simulink model "control_demo"  (R2022a)
settings: Solver=FixedStepAuto  StartTime=0.0  StopTime=10  FixedStep=Ts  RelTol=1e-3
values from neighbouring files (symbols this model uses):
  fil = 0.1    [Decen_control_prepare.m]    (also in control_demo_prepare.m = 0.0001; simulation_CPG.m = 0.0001)
  K_a = diag([0.001,0.001])    [control_demo_prepare.m]
  K_d = diag([5,5])    [control_demo_prepare.m]    (also in simulation_CPG.m)
  K_p = diag([1000,1000])    [control_demo_prepare.m]    (also in simulation_CPG.m)
  Tc = 0.001    [Decen_control_prepare.m]    (also in control_demo_prepare.m; simulation_CPG.m)
undefined symbols (not defined in the file or in its folder): duration, effort, IFV, index, iner, joint_name, LF_body2thigh, LF_thigh2calf, LH_body2thigh, LH_thigh2calf, model_name, RF_body2thigh, RF_thigh2calf, RH_body2thigh, RH_thigh2calf
libraries: robotgazebolib x27
settings Model: PauseTimes=2  Creator=liltrump  LastModifiedBy=liltrump

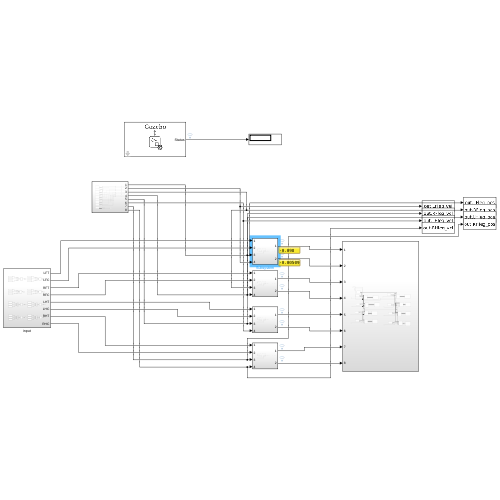
[thumbnail: Simulink's stored preview of the top-level diagram]
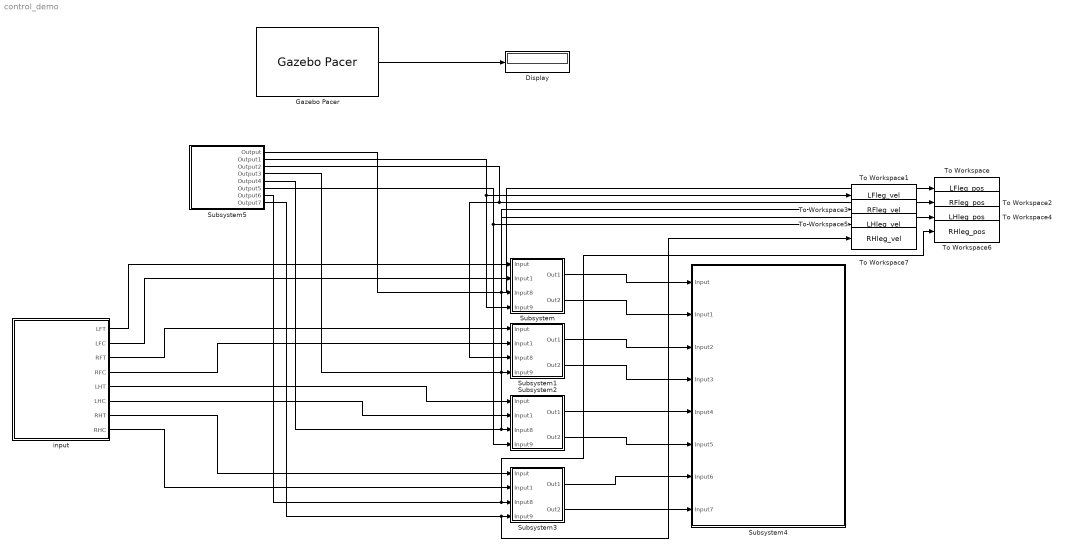
== system control_demo ==
  Display : Display
  Gazebo Pacer : robotgazebolib/Gazebo Pacer  ResetBehavior=Reset Gazebo simulation time and scene  SampleTime=0.001
      settings: SourceProductBaseCode=RO
  Subsystem : Subsystem
  Subsystem1 : Subsystem
  Subsystem2 : Subsystem
  Subsystem3 : Subsystem
  Subsystem4 : Subsystem
  Subsystem5 : Subsystem
  To Workspace : ToWorkspace  VariableName=LFleg_pos  SaveFormat=Timeseries  SampleTime=-1
  To Workspace1 : ToWorkspace  VariableName=LFleg_vel  SaveFormat=Timeseries  SampleTime=-1
  To Workspace2 : ToWorkspace  VariableName=RFleg_pos  SaveFormat=Timeseries  SampleTime=-1
  To Workspace3 : ToWorkspace  VariableName=RFleg_vel  SaveFormat=Timeseries  SampleTime=-1
  To Workspace4 : ToWorkspace  VariableName=LHleg_pos  SaveFormat=Timeseries  SampleTime=-1
  To Workspace5 : ToWorkspace  VariableName=LHleg_vel  SaveFormat=Timeseries  SampleTime=-1
  To Workspace6 : ToWorkspace  VariableName=RHleg_pos  SaveFormat=Timeseries  SampleTime=-1
  To Workspace7 : ToWorkspace  VariableName=RHleg_vel  SaveFormat=Timeseries  SampleTime=-1
  input : Subsystem
  wires:
  Gazebo Pacer/1 -> Display/1
  Subsystem5/1(Output) -> To Workspace/1, Subsystem/3(Input8)
  Subsystem5/2(Output1) -> To Workspace1/1, Subsystem/4(Input9)
  Subsystem5/3(Output2) -> Subsystem1/3(Input8), To Workspace2/1
  Subsystem5/4(Output3) -> Subsystem1/4(Input9), To Workspace3/1
  Subsystem5/5(Output4) -> Subsystem2/3(Input8), To Workspace4/1
  Subsystem5/6(Output5) -> Subsystem2/4(Input9), To Workspace5/1
  Subsystem5/7(Output6) -> Subsystem3/3(Input8), To Workspace6/1
  Subsystem5/8(Output7) -> Subsystem3/4(Input9), To Workspace7/1
  Subsystem/1(Out1) -> Subsystem4/1(Input)
  Subsystem/2(Out2) -> Subsystem4/2(Input1)
  Subsystem1/1(Out1) -> Subsystem4/3(Input2)
  Subsystem1/2(Out2) -> Subsystem4/4(Input3)
  Subsystem2/1(Out1) -> Subsystem4/5(Input4)
  Subsystem2/2(Out2) -> Subsystem4/6(Input5)
  Subsystem3/1(Out1) -> Subsystem4/7(Input6)
  Subsystem3/2(Out2) -> Subsystem4/8(Input7)
  input/1(LFT) -> Subsystem/1(Input)
  input/2(LFC) -> Subsystem/2(Input1)
  input/3(RFT) -> Subsystem1/1(Input)
  input/4(RFC) -> Subsystem1/2(Input1)
  input/5(LHT) -> Subsystem2/1(Input)
  input/6(LHC) -> Subsystem2/2(Input1)
  input/7(RHT) -> Subsystem3/1(Input)
  input/8(RHC) -> Subsystem3/2(Input1)

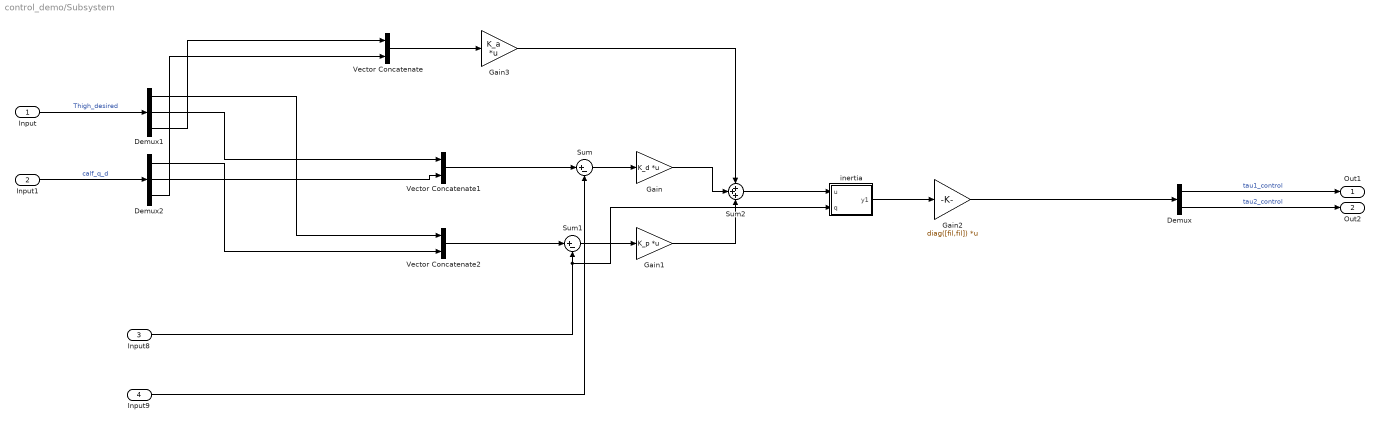
== system control_demo/Subsystem ==
  Input : Inport
  Input1 : Inport  Port=2
  Input8 : Inport  Port=3
  Input9 : Inport  Port=4
  Demux : Demux  Outputs=2
  Demux1 : Demux  Outputs=3
  Demux2 : Demux  Outputs=3
  Gain : Gain  Gain=K_d  Multiplication=Matrix(K*u)
  Gain1 : Gain  Gain=K_p  Multiplication=Matrix(K*u)
  Gain2 : Gain  Gain=diag([fil,fil])  Multiplication=Matrix(K*u)
  Gain3 : Gain  Gain=K_a  Multiplication=Matrix(K*u)
  Sum : Sum  Inputs=|+-
  Sum1 : Sum  Inputs=|+-
  Sum2 : Sum  Inputs=+++
  Vector Concatenate : Concatenate
  Vector Concatenate1 : Concatenate
  Vector Concatenate2 : Concatenate
  inertia : Subsystem
      mask Display: disp('B(q)u')
  Out1 : Outport
  Out2 : Outport  Port=2
  wires:
  Gain1/1 -> Sum2/3
  Vector Concatenate1/1 -> Sum/1
  Sum/1 -> Gain/1
  Sum2/1 -> inertia/1(u)
  Sum1/1 -> Gain1/1
  Gain/1 -> Sum2/2
  Vector Concatenate2/1 -> Sum1/1
  Input8/1 -> inertia/2(q), Sum1/2
  Input9/1 -> Sum/2
  Demux/2 -> Out2/1  "tau2_control"
  Demux/1 -> Out1/1  "tau1_control"
  inertia/1(y1) -> Gain2/1
  Gain2/1 -> Demux/1
  Input/1 -> Demux1/1  "Thigh_desired"
  Input1/1 -> Demux2/1  "calf_q_d"
  Demux1/1 -> Vector Concatenate2/1
  Demux2/1 -> Vector Concatenate2/2
  Demux1/2 -> Vector Concatenate1/1
  Demux2/2 -> Vector Concatenate1/2
  Demux1/3 -> Vector Concatenate/1
  Demux2/3 -> Vector Concatenate/2
  Vector Concatenate/1 -> Gain3/1
  Gain3/1 -> Sum2/1

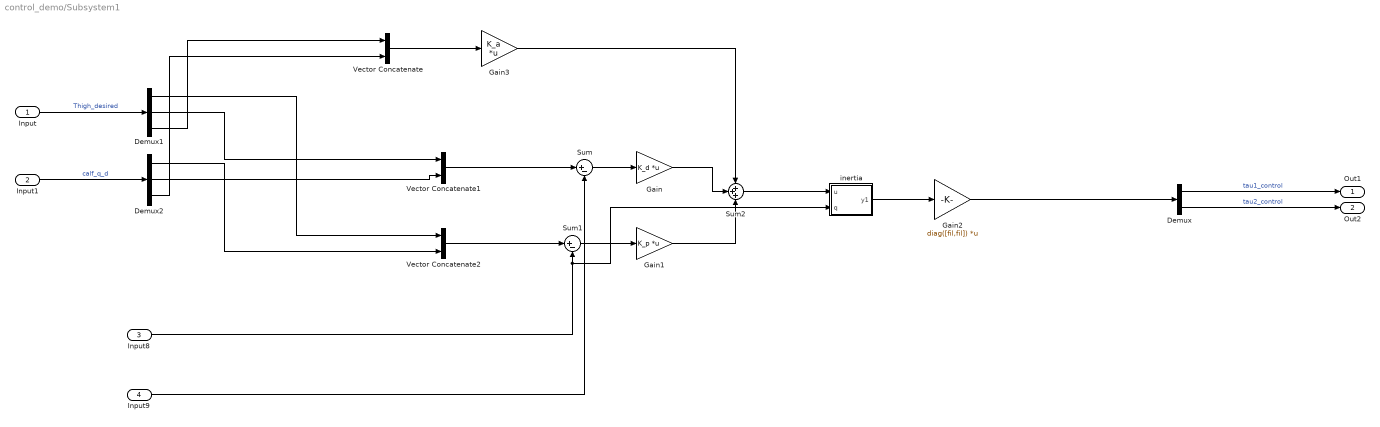
== system control_demo/Subsystem1 ==
  Input : Inport
  Input1 : Inport  Port=2
  Input8 : Inport  Port=3
  Input9 : Inport  Port=4
  Demux : Demux  Outputs=2
  Demux1 : Demux  Outputs=3
  Demux2 : Demux  Outputs=3
  Gain : Gain  Gain=K_d  Multiplication=Matrix(K*u)
  Gain1 : Gain  Gain=K_p  Multiplication=Matrix(K*u)
  Gain2 : Gain  Gain=diag([fil,fil])  Multiplication=Matrix(K*u)
  Gain3 : Gain  Gain=K_a  Multiplication=Matrix(K*u)
  Sum : Sum  Inputs=|+-
  Sum1 : Sum  Inputs=|+-
  Sum2 : Sum  Inputs=+++
  Vector Concatenate : Concatenate
  Vector Concatenate1 : Concatenate
  Vector Concatenate2 : Concatenate
  inertia : Subsystem
      mask Display: disp('B(q)u')
  Out1 : Outport
  Out2 : Outport  Port=2
  wires:
  Gain1/1 -> Sum2/3
  Vector Concatenate1/1 -> Sum/1
  Sum/1 -> Gain/1
  Sum2/1 -> inertia/1(u)
  Sum1/1 -> Gain1/1
  Gain/1 -> Sum2/2
  Vector Concatenate2/1 -> Sum1/1
  Input8/1 -> inertia/2(q), Sum1/2
  Input9/1 -> Sum/2
  Demux/2 -> Out2/1  "tau2_control"
  Demux/1 -> Out1/1  "tau1_control"
  inertia/1(y1) -> Gain2/1
  Gain2/1 -> Demux/1
  Input/1 -> Demux1/1  "Thigh_desired"
  Input1/1 -> Demux2/1  "calf_q_d"
  Demux1/1 -> Vector Concatenate2/1
  Demux2/1 -> Vector Concatenate2/2
  Demux1/2 -> Vector Concatenate1/1
  Demux2/2 -> Vector Concatenate1/2
  Demux1/3 -> Vector Concatenate/1
  Demux2/3 -> Vector Concatenate/2
  Vector Concatenate/1 -> Gain3/1
  Gain3/1 -> Sum2/1

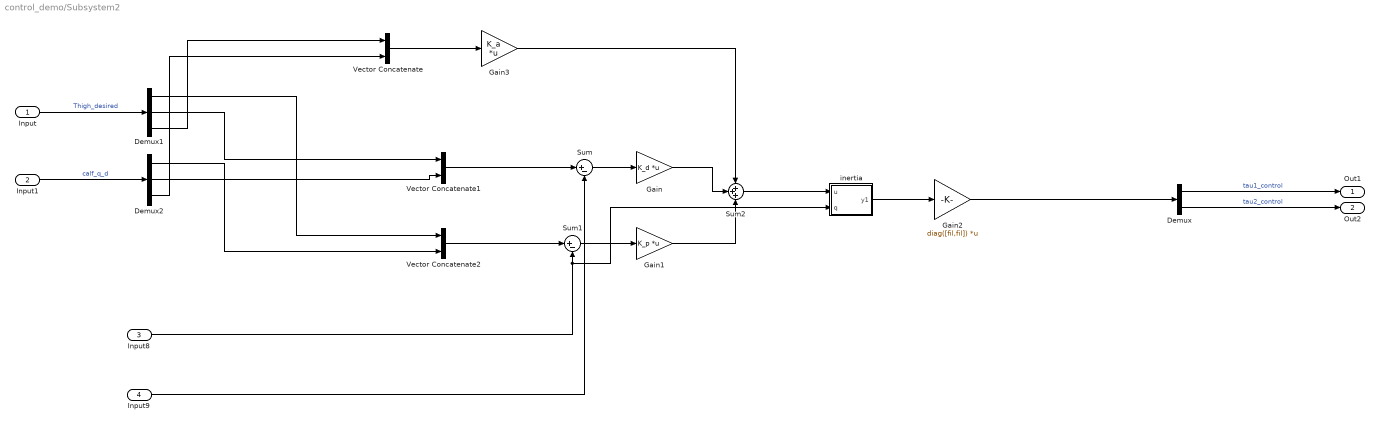
== system control_demo/Subsystem2 ==
  Input : Inport
  Input1 : Inport  Port=2
  Input8 : Inport  Port=3
  Input9 : Inport  Port=4
  Demux : Demux  Outputs=2
  Demux1 : Demux  Outputs=3
  Demux2 : Demux  Outputs=3
  Gain : Gain  Gain=K_d  Multiplication=Matrix(K*u)
  Gain1 : Gain  Gain=K_p  Multiplication=Matrix(K*u)
  Gain2 : Gain  Gain=diag([fil,fil])  Multiplication=Matrix(K*u)
  Gain3 : Gain  Gain=K_a  Multiplication=Matrix(K*u)
  Sum : Sum  Inputs=|+-
  Sum1 : Sum  Inputs=|+-
  Sum2 : Sum  Inputs=+++
  Vector Concatenate : Concatenate
  Vector Concatenate1 : Concatenate
  Vector Concatenate2 : Concatenate
  inertia : Subsystem
      mask Display: disp('B(q)u')
  Out1 : Outport
  Out2 : Outport  Port=2
  wires:
  Gain1/1 -> Sum2/3
  Vector Concatenate1/1 -> Sum/1
  Sum/1 -> Gain/1
  Sum2/1 -> inertia/1(u)
  Sum1/1 -> Gain1/1
  Gain/1 -> Sum2/2
  Vector Concatenate2/1 -> Sum1/1
  Input8/1 -> inertia/2(q), Sum1/2
  Input9/1 -> Sum/2
  Demux/2 -> Out2/1  "tau2_control"
  Demux/1 -> Out1/1  "tau1_control"
  inertia/1(y1) -> Gain2/1
  Gain2/1 -> Demux/1
  Input/1 -> Demux1/1  "Thigh_desired"
  Input1/1 -> Demux2/1  "calf_q_d"
  Demux1/1 -> Vector Concatenate2/1
  Demux2/1 -> Vector Concatenate2/2
  Demux1/2 -> Vector Concatenate1/1
  Demux2/2 -> Vector Concatenate1/2
  Demux1/3 -> Vector Concatenate/1
  Demux2/3 -> Vector Concatenate/2
  Vector Concatenate/1 -> Gain3/1
  Gain3/1 -> Sum2/1

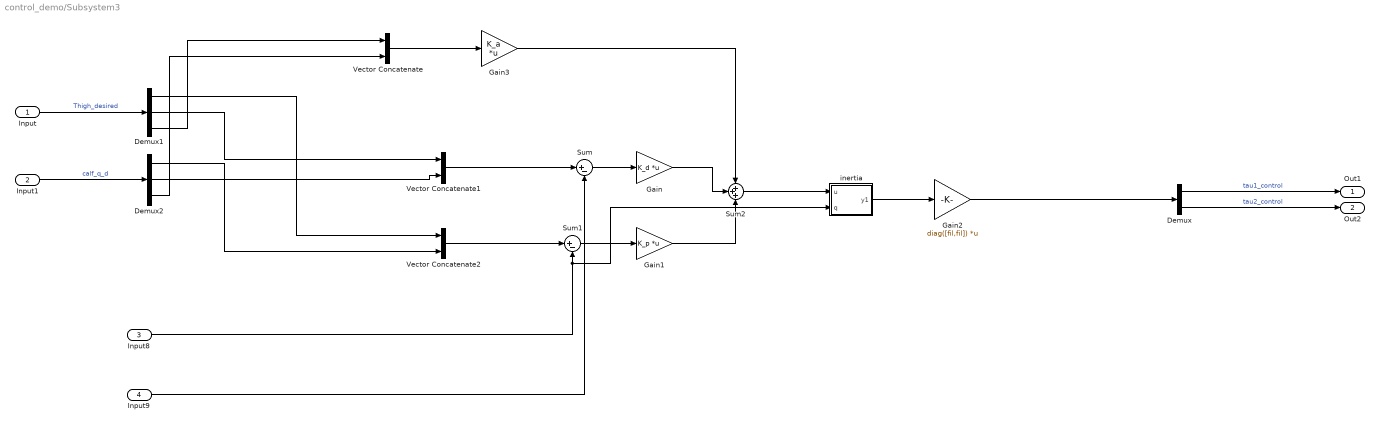
== system control_demo/Subsystem3 ==
  Input : Inport
  Input1 : Inport  Port=2
  Input8 : Inport  Port=3
  Input9 : Inport  Port=4
  Demux : Demux  Outputs=2
  Demux1 : Demux  Outputs=3
  Demux2 : Demux  Outputs=3
  Gain : Gain  Gain=K_d  Multiplication=Matrix(K*u)
  Gain1 : Gain  Gain=K_p  Multiplication=Matrix(K*u)
  Gain2 : Gain  Gain=diag([fil,fil])  Multiplication=Matrix(K*u)
  Gain3 : Gain  Gain=K_a  Multiplication=Matrix(K*u)
  Sum : Sum  Inputs=|+-
  Sum1 : Sum  Inputs=|+-
  Sum2 : Sum  Inputs=+++
  Vector Concatenate : Concatenate
  Vector Concatenate1 : Concatenate
  Vector Concatenate2 : Concatenate
  inertia : Subsystem
      mask Display: disp('B(q)u')
  Out1 : Outport
  Out2 : Outport  Port=2
  wires:
  Gain1/1 -> Sum2/3
  Vector Concatenate1/1 -> Sum/1
  Sum/1 -> Gain/1
  Sum2/1 -> inertia/1(u)
  Sum1/1 -> Gain1/1
  Gain/1 -> Sum2/2
  Vector Concatenate2/1 -> Sum1/1
  Input8/1 -> inertia/2(q), Sum1/2
  Input9/1 -> Sum/2
  Demux/2 -> Out2/1  "tau2_control"
  Demux/1 -> Out1/1  "tau1_control"
  inertia/1(y1) -> Gain2/1
  Gain2/1 -> Demux/1
  Input/1 -> Demux1/1  "Thigh_desired"
  Input1/1 -> Demux2/1  "calf_q_d"
  Demux1/1 -> Vector Concatenate2/1
  Demux2/1 -> Vector Concatenate2/2
  Demux1/2 -> Vector Concatenate1/1
  Demux2/2 -> Vector Concatenate1/2
  Demux1/3 -> Vector Concatenate/1
  Demux2/3 -> Vector Concatenate/2
  Vector Concatenate/1 -> Gain3/1
  Gain3/1 -> Sum2/1

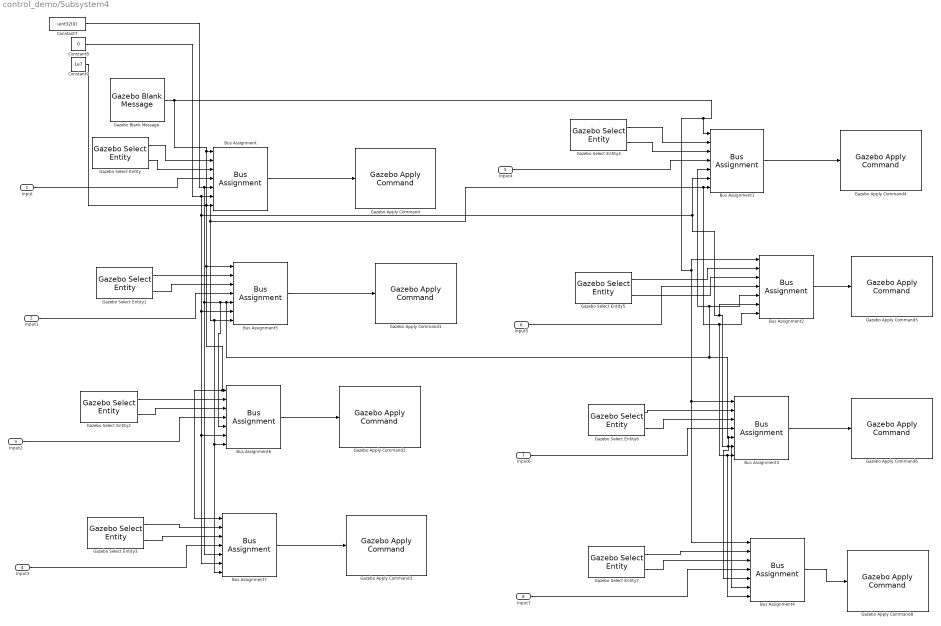
== system control_demo/Subsystem4 ==
  Input : Inport
  Input1 : Inport  Port=2
  Input2 : Inport  Port=3
  Input3 : Inport  Port=4
  Input4 : Inport  Port=5
  Input5 : Inport  Port=6
  Input6 : Inport  Port=7
  Input7 : Inport  Port=8
  Bus Assignment{,1..7} (8 alike) : BusAssignment  AssignedSignals=model_name,joint_name,effort,index,duration.seconds,duration.nano_seconds
  Constant7 : Constant  Value=uint32(0)
  Constant8 : Constant  Value=0
  Constant9 : Constant  Value=1e7
  Gazebo Apply Command{,1..6,8} (8 alike) : robotgazebolib/Gazebo Apply Command  cmdType=ApplyJointTorque  sampleTime=0.001
      settings: SourceProductBaseCode=RO
  Gazebo Blank Message : robotgazebolib/Gazebo Blank Message  msgType=ApplyJointTorque  sampleTime=0.001  busName='Gazebo_SL_Bus_gazebo_msgs_ApplyJointTorque'
      settings: SourceProductBaseCode=RO
  Gazebo Select Entity : robotgazebolib/Gazebo Select Entity  modelElemName=IFV/LF_body2thigh  outputArraySize=128  OutputLabel=Joint  SelectType=Joint
      settings: SourceProductBaseCode=RO
  Gazebo Select Entity1 : robotgazebolib/Gazebo Select Entity  modelElemName=IFV/LF_thigh2calf  outputArraySize=128  OutputLabel=Joint  SelectType=Joint
      settings: SourceProductBaseCode=RO
  Gazebo Select Entity2 : robotgazebolib/Gazebo Select Entity  modelElemName=IFV/RF_body2thigh  outputArraySize=128  OutputLabel=Joint  SelectType=Joint
      settings: SourceProductBaseCode=RO
  Gazebo Select Entity3 : robotgazebolib/Gazebo Select Entity  modelElemName=IFV/RF_thigh2calf  outputArraySize=128  OutputLabel=Joint  SelectType=Joint
      settings: SourceProductBaseCode=RO
  Gazebo Select Entity4 : robotgazebolib/Gazebo Select Entity  modelElemName=IFV/LH_body2thigh  outputArraySize=128  OutputLabel=Joint  SelectType=Joint
      settings: SourceProductBaseCode=RO
  Gazebo Select Entity5 : robotgazebolib/Gazebo Select Entity  modelElemName=IFV/LH_thigh2calf  outputArraySize=128  OutputLabel=Joint  SelectType=Joint
      settings: SourceProductBaseCode=RO
  Gazebo Select Entity6 : robotgazebolib/Gazebo Select Entity  modelElemName=IFV/RH_body2thigh  outputArraySize=128  OutputLabel=Joint  SelectType=Joint
      settings: SourceProductBaseCode=RO
  Gazebo Select Entity7 : robotgazebolib/Gazebo Select Entity  modelElemName=IFV/RH_thigh2calf  outputArraySize=128  OutputLabel=Joint  SelectType=Joint
      settings: SourceProductBaseCode=RO
  wires:
  Gazebo Select Entity/1 -> Bus Assignment/2
  Gazebo Select Entity/2 -> Bus Assignment/3
  Bus Assignment/1 -> Gazebo Apply Command/1
  Input/1 -> Bus Assignment/4
  Bus Assignment5/1 -> Gazebo Apply Command1/1
  Input1/1 -> Bus Assignment5/4
  Gazebo Select Entity1/1 -> Bus Assignment5/2
  Gazebo Select Entity1/2 -> Bus Assignment5/3
  Bus Assignment6/1 -> Gazebo Apply Command2/1
  Input2/1 -> Bus Assignment6/4
  Gazebo Select Entity2/1 -> Bus Assignment6/2
  Gazebo Select Entity2/2 -> Bus Assignment6/3
  Bus Assignment7/1 -> Gazebo Apply Command3/1
  Input3/1 -> Bus Assignment7/4
  Gazebo Select Entity3/1 -> Bus Assignment7/2
  Gazebo Select Entity3/2 -> Bus Assignment7/3
  Bus Assignment1/1 -> Gazebo Apply Command4/1
  Gazebo Select Entity4/1 -> Bus Assignment1/2
  Gazebo Select Entity4/2 -> Bus Assignment1/3
  Bus Assignment2/1 -> Gazebo Apply Command5/1
  Gazebo Select Entity5/1 -> Bus Assignment2/2
  Gazebo Select Entity5/2 -> Bus Assignment2/3
  Bus Assignment3/1 -> Gazebo Apply Command6/1
  Input6/1 -> Bus Assignment3/4
  Gazebo Select Entity6/1 -> Bus Assignment3/2
  Gazebo Select Entity6/2 -> Bus Assignment3/3
  Bus Assignment4/1 -> Gazebo Apply Command8/1
  Input7/1 -> Bus Assignment4/4
  Gazebo Select Entity7/1 -> Bus Assignment4/2
  Gazebo Blank Message/1 -> Bus Assignment1/1, Bus Assignment2/1, Bus Assignment4/1, Bus Assignment3/1, Bus Assignment5/1, Bus Assignment7/1, Bus Assignment6/1, Bus Assignment/1
  Gazebo Select Entity7/2 -> Bus Assignment4/3
  Constant7/1 -> Bus Assignment/5, Bus Assignment6/5, Bus Assignment4/5, Bus Assignment3/5, Bus Assignment1/5, Bus Assignment2/5, Bus Assignment5/5, Bus Assignment7/5
  Constant8/1 -> Bus Assignment7/6, Bus Assignment6/6, Bus Assignment5/6, Bus Assignment4/6, Bus Assignment3/6, Bus Assignment2/6, Bus Assignment1/6, Bus Assignment/6
  Constant9/1 -> Bus Assignment5/7, Bus Assignment7/7, Bus Assignment6/7, Bus Assignment4/7, Bus Assignment3/7, Bus Assignment2/7, Bus Assignment1/7, Bus Assignment/7
  Input4/1 -> Bus Assignment1/4
  Input5/1 -> Bus Assignment2/4

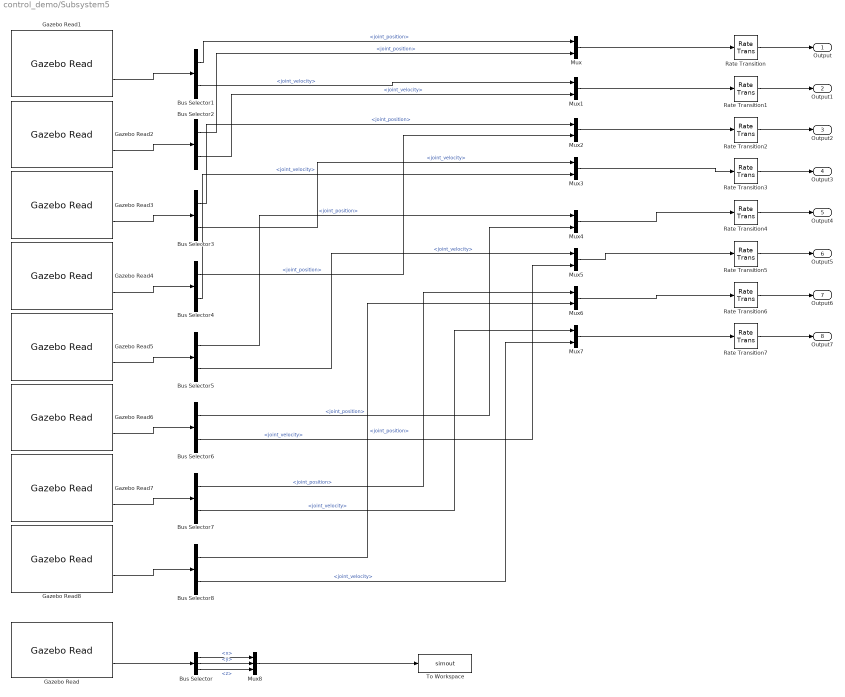
== system control_demo/Subsystem5 ==
  Bus Selector : BusSelector  OutputSignals=world_linear_velocity.x,world_linear_velocity.y,world_linear_velocity.z
  Bus Selector{1..8} (8 alike) : BusSelector  OutputSignals=joint_position,joint_velocity
  Gazebo Read : robotgazebolib/Gazebo Read  topicSource=From Gazebo  topic=/gazebo/ground_truth/link_state/IFV/chassis  messageType=gazebo_msgs/LinkState  sampleTime=0.001
      settings: SourceProductBaseCode=RO
  Gazebo Read1 : robotgazebolib/Gazebo Read  topicSource=From Gazebo  topic=/gazebo/ground_truth/joint_state/IFV/LF_body2thigh  messageType=gazebo_msgs/JointState  sampleTime=0.001
      settings: SourceProductBaseCode=RO
  Gazebo Read2 : robotgazebolib/Gazebo Read  topicSource=From Gazebo  topic=/gazebo/ground_truth/joint_state/IFV/LF_thigh2calf  messageType=gazebo_msgs/JointState  sampleTime=0.001
      settings: SourceProductBaseCode=RO
  Gazebo Read3 : robotgazebolib/Gazebo Read  topicSource=From Gazebo  topic=/gazebo/ground_truth/joint_state/IFV/RF_body2thigh  messageType=gazebo_msgs/JointState  sampleTime=0.001
      settings: SourceProductBaseCode=RO
  Gazebo Read4 : robotgazebolib/Gazebo Read  topicSource=From Gazebo  topic=/gazebo/ground_truth/joint_state/IFV/RF_thigh2calf  messageType=gazebo_msgs/JointState  sampleTime=0.001
      settings: SourceProductBaseCode=RO
  Gazebo Read5 : robotgazebolib/Gazebo Read  topicSource=From Gazebo  topic=/gazebo/ground_truth/joint_state/IFV/LH_body2thigh  messageType=gazebo_msgs/JointState  sampleTime=0.001
      settings: SourceProductBaseCode=RO
  Gazebo Read6 : robotgazebolib/Gazebo Read  topicSource=From Gazebo  topic=/gazebo/ground_truth/joint_state/IFV/LH_thigh2calf  messageType=gazebo_msgs/JointState  sampleTime=0.001
      settings: SourceProductBaseCode=RO
  Gazebo Read7 : robotgazebolib/Gazebo Read  topicSource=From Gazebo  topic=/gazebo/ground_truth/joint_state/IFV/RH_body2thigh  messageType=gazebo_msgs/JointState  sampleTime=0.001
      settings: SourceProductBaseCode=RO
  Gazebo Read8 : robotgazebolib/Gazebo Read  topicSource=From Gazebo  topic=/gazebo/ground_truth/joint_state/IFV/RH_thigh2calf  messageType=gazebo_msgs/JointState  sampleTime=0.001
      settings: SourceProductBaseCode=RO
  Mux{,1..7} (8 alike) : Mux  Inputs=2
  Mux8 : Mux  Inputs=3
  Rate Transition{,1..7} (8 alike) : RateTransition
  To Workspace : ToWorkspace  VariableName=simout  SaveFormat=Timeseries  SampleTime=-1
  Output : Outport
  Output1 : Outport  Port=2
  Output2 : Outport  Port=3
  Output3 : Outport  Port=4
  Output4 : Outport  Port=5
  Output5 : Outport  Port=6
  Output6 : Outport  Port=7
  Output7 : Outport  Port=8
  wires:
  Gazebo Read1/2 -> Bus Selector1/1
  Bus Selector2/2 -> Mux1/2  "<joint_velocity>"
  Gazebo Read2/2 -> Bus Selector2/1
  Gazebo Read3/2 -> Bus Selector3/1
  Gazebo Read4/2 -> Bus Selector4/1
  Gazebo Read5/2 -> Bus Selector5/1
  Gazebo Read6/2 -> Bus Selector6/1
  Gazebo Read7/2 -> Bus Selector7/1
  Gazebo Read8/2 -> Bus Selector8/1
  Mux1/1 -> Rate Transition1/1
  Mux2/1 -> Rate Transition2/1
  Mux3/1 -> Rate Transition3/1
  Mux4/1 -> Rate Transition4/1
  Mux5/1 -> Rate Transition5/1
  Mux6/1 -> Rate Transition6/1
  Mux7/1 -> Rate Transition7/1
  Bus Selector1/2 -> Mux1/1  "<joint_velocity>"
  Bus Selector1/1 -> Mux/1  "<joint_position>"
  Bus Selector2/1 -> Mux/2  "<joint_position>"
  Mux/1 -> Rate Transition/1
  Rate Transition/1 -> Output/1
  Rate Transition1/1 -> Output1/1
  Rate Transition2/1 -> Output2/1
  Rate Transition3/1 -> Output3/1
  Rate Transition4/1 -> Output4/1
  Rate Transition5/1 -> Output5/1
  Rate Transition6/1 -> Output6/1
  Rate Transition7/1 -> Output7/1
  Bus Selector3/1 -> Mux2/1  "<joint_position>"
  Bus Selector4/1 -> Mux2/2  "<joint_position>"
  Bus Selector3/2 -> Mux3/1  "<joint_velocity>"
  Bus Selector4/2 -> Mux3/2  "<joint_velocity>"
  Bus Selector5/1 -> Mux4/1  "<joint_position>"
  Bus Selector6/1 -> Mux4/2  "<joint_position>"
  Bus Selector5/2 -> Mux5/1  "<joint_velocity>"
  Bus Selector6/2 -> Mux5/2  "<joint_velocity>"
  Bus Selector7/1 -> Mux6/1  "<joint_position>"
  Bus Selector7/2 -> Mux7/1  "<joint_velocity>"
  Bus Selector8/1 -> Mux6/2  "<joint_position>"
  Bus Selector8/2 -> Mux7/2  "<joint_velocity>"
  Gazebo Read/2 -> Bus Selector/1
  Bus Selector/1 -> Mux8/1  "<x>"
  Bus Selector/3 -> Mux8/3  "<z>"
  Mux8/1 -> To Workspace/1
  Bus Selector/2 -> Mux8/2  "<y>"

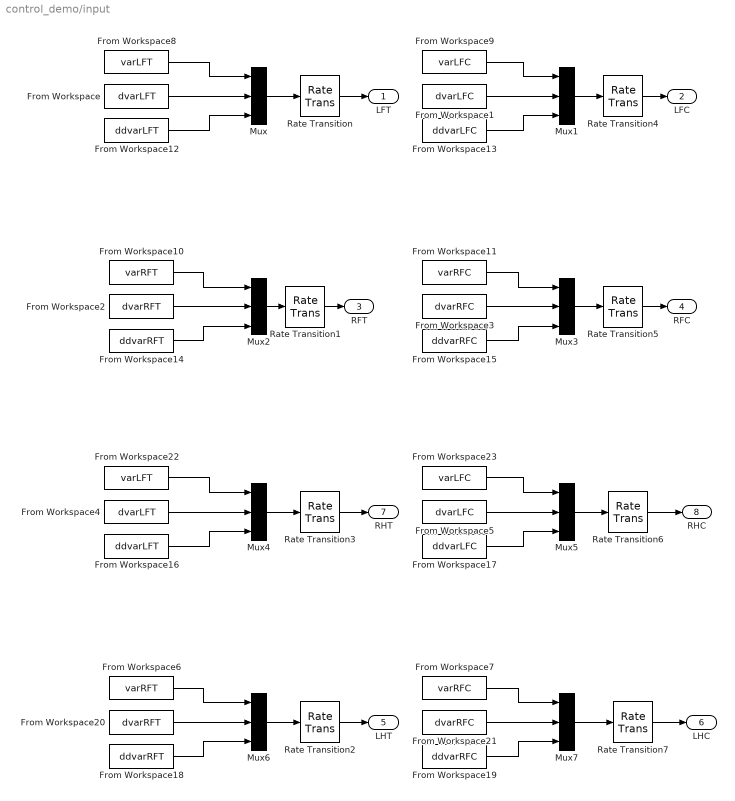
== system control_demo/input ==
  From Workspace : FromWorkspace  VariableName=dvarLFT
  From Workspace1 : FromWorkspace  VariableName=dvarLFC
  From Workspace10 : FromWorkspace  VariableName=varRFT
  From Workspace11 : FromWorkspace  VariableName=varRFC
  From Workspace12 : FromWorkspace  VariableName=ddvarLFT
  From Workspace13 : FromWorkspace  VariableName=ddvarLFC
  From Workspace14 : FromWorkspace  VariableName=ddvarRFT
  From Workspace15 : FromWorkspace  VariableName=ddvarRFC
  From Workspace16 : FromWorkspace  VariableName=ddvarLFT
  From Workspace17 : FromWorkspace  VariableName=ddvarLFC
  From Workspace18 : FromWorkspace  VariableName=ddvarRFT
  From Workspace19 : FromWorkspace  VariableName=ddvarRFC
  From Workspace2 : FromWorkspace  VariableName=dvarRFT
  From Workspace20 : FromWorkspace  VariableName=dvarRFT
  From Workspace21 : FromWorkspace  VariableName=dvarRFC
  From Workspace22 : FromWorkspace  VariableName=varLFT
  From Workspace23 : FromWorkspace  VariableName=varLFC
  From Workspace3 : FromWorkspace  VariableName=dvarRFC
  From Workspace4 : FromWorkspace  VariableName=dvarLFT
  From Workspace5 : FromWorkspace  VariableName=dvarLFC
  From Workspace6 : FromWorkspace  VariableName=varRFT
  From Workspace7 : FromWorkspace  VariableName=varRFC
  From Workspace8 : FromWorkspace  VariableName=varLFT  OutputAfterFinalValue=Setting to zero
  From Workspace9 : FromWorkspace  VariableName=varLFC
  Mux{,1..7} (8 alike) : Mux  Inputs=3
  Rate Transition{,1..7} (8 alike) : RateTransition
  LFT : Outport
  LFC : Outport  Port=2
  RFT : Outport  Port=3
  RFC : Outport  Port=4
  LHT : Outport  Port=5
  LHC : Outport  Port=6
  RHT : Outport  Port=7
  RHC : Outport  Port=8
  wires:
  From Workspace8/1 -> Mux/1
  From Workspace/1 -> Mux/2
  From Workspace12/1 -> Mux/3
  From Workspace10/1 -> Mux2/1
  From Workspace2/1 -> Mux2/2
  From Workspace14/1 -> Mux2/3
  From Workspace9/1 -> Mux1/1
  From Workspace1/1 -> Mux1/2
  From Workspace13/1 -> Mux1/3
  From Workspace11/1 -> Mux3/1
  From Workspace3/1 -> Mux3/2
  From Workspace15/1 -> Mux3/3
  Mux1/1 -> Rate Transition4/1
  Mux2/1 -> Rate Transition1/1
  Mux3/1 -> Rate Transition5/1
  From Workspace6/1 -> Mux6/1
  From Workspace19/1 -> Mux7/3
  From Workspace20/1 -> Mux6/2
  Mux4/1 -> Rate Transition3/1
  From Workspace5/1 -> Mux5/2
  From Workspace17/1 -> Mux5/3
  From Workspace21/1 -> Mux7/2
  From Workspace22/1 -> Mux4/1
  Mux5/1 -> Rate Transition6/1
  From Workspace18/1 -> Mux6/3
  From Workspace23/1 -> Mux5/1
  From Workspace16/1 -> Mux4/3
  Mux7/1 -> Rate Transition7/1
  Mux6/1 -> Rate Transition2/1
  From Workspace7/1 -> Mux7/1
  From Workspace4/1 -> Mux4/2
  Mux/1 -> Rate Transition/1
  Rate Transition/1 -> LFT/1
  Rate Transition1/1 -> RFT/1
  Rate Transition2/1 -> LHT/1
  Rate Transition3/1 -> RHT/1
  Rate Transition4/1 -> LFC/1
  Rate Transition5/1 -> RFC/1
  Rate Transition6/1 -> RHC/1
  Rate Transition7/1 -> LHC/1

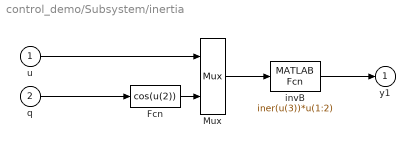
== system control_demo/Subsystem/inertia ==
  u : Inport
  q : Inport  Port=2
  Fcn : Fcn  Expr=cos(u(2))  SampleTime=Tc
  Mux : Mux  Inputs=[2,1]
  "invB " : MATLABFcn  MATLABFcn=iner(u(3))*u(1:2)  OutputDimensions=2  OutputSignalType=real  SampleTime=Tc
      mask Display: disp('B(q)')
  y1 : Outport  InitialOutput=0
  wires:
  u/1 -> Mux/1
  q/1 -> Fcn/1
  Mux/1 -> "invB "/1
  "invB "/1 -> y1/1
  Fcn/1 -> Mux/2

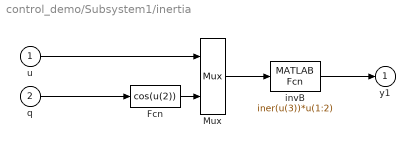
== system control_demo/Subsystem1/inertia ==
  u : Inport
  q : Inport  Port=2
  Fcn : Fcn  Expr=cos(u(2))  SampleTime=Tc
  Mux : Mux  Inputs=[2,1]
  "invB " : MATLABFcn  MATLABFcn=iner(u(3))*u(1:2)  OutputDimensions=2  OutputSignalType=real  SampleTime=Tc
      mask Display: disp('B(q)')
  y1 : Outport  InitialOutput=0
  wires:
  u/1 -> Mux/1
  q/1 -> Fcn/1
  Mux/1 -> "invB "/1
  "invB "/1 -> y1/1
  Fcn/1 -> Mux/2

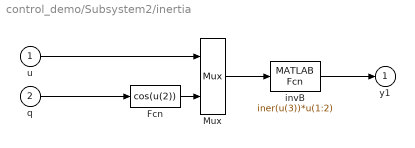
== system control_demo/Subsystem2/inertia ==
  u : Inport
  q : Inport  Port=2
  Fcn : Fcn  Expr=cos(u(2))  SampleTime=Tc
  Mux : Mux  Inputs=[2,1]
  "invB " : MATLABFcn  MATLABFcn=iner(u(3))*u(1:2)  OutputDimensions=2  OutputSignalType=real  SampleTime=Tc
      mask Display: disp('B(q)')
  y1 : Outport  InitialOutput=0
  wires:
  u/1 -> Mux/1
  q/1 -> Fcn/1
  Mux/1 -> "invB "/1
  "invB "/1 -> y1/1
  Fcn/1 -> Mux/2

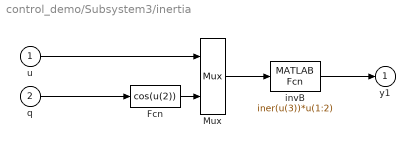
== system control_demo/Subsystem3/inertia ==
  u : Inport
  q : Inport  Port=2
  Fcn : Fcn  Expr=cos(u(2))  SampleTime=Tc
  Mux : Mux  Inputs=[2,1]
  "invB " : MATLABFcn  MATLABFcn=iner(u(3))*u(1:2)  OutputDimensions=2  OutputSignalType=real  SampleTime=Tc
      mask Display: disp('B(q)')
  y1 : Outport  InitialOutput=0
  wires:
  u/1 -> Mux/1
  q/1 -> Fcn/1
  Mux/1 -> "invB "/1
  "invB "/1 -> y1/1
  Fcn/1 -> Mux/2
